simulink model "V3_sim"  (R2017a)
settings: Solver=ode45  StartTime=0.0  StopTime=Te-1  RelTol=1e-10  EnableMultiTasking=on
InitFcn:
  | clear persistent;
  | initScript;
values from neighbouring files (symbols this model uses):
  stPendel = ladePendel()    [V6_main.m]    (also in initScript.m)
  stTraj =     [Copy_of_traj.mat]    (also in traj.mat)
  T_M = .01    (= 0.01)    [initScript.m]
  x0 = [0 0 0 0]'    [RandwertproblemStates.m]    (also in initScript.m = [0 0 0 0])
settings Model: Creator=bened  LastModifiedBy=bened
settings OptimizationCC: LifeSpan=inf
settings DebuggingCC: SFUnexpectedBacktrackingDiag=warning  SFNoUnconditionalDefaultTransitionDiag=warning  SFExecutionAtInitializationDiag=none
settings GRTTargetCC: TargetLangStandard=C89/C90 (ANSI)
settings ConfigComp: CovMetricSettings=dw  CovHtmlReporting=on  CovSaveCumulativeToWorkspaceVar=on  CovSaveSingleToWorkspaceVar=on  CovExternalEMLEnable=off

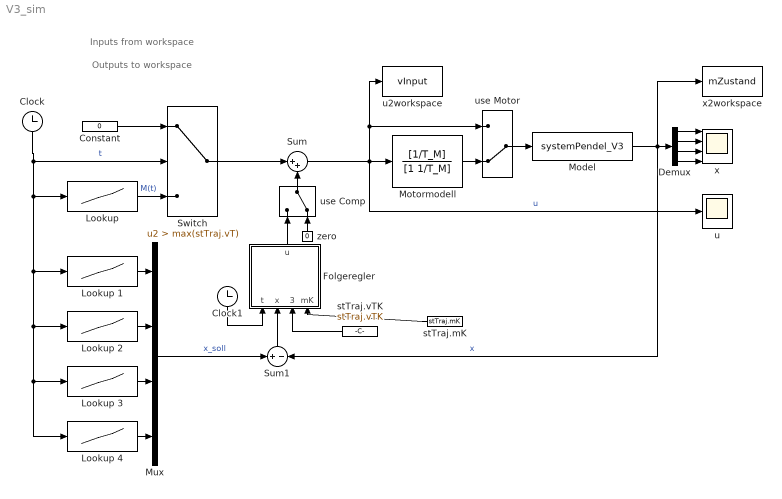
== system V3_sim ==
  note: Inputs from workspace
  note: Outputs to workspace
  Clock : Clock
  Clock1 : Clock
  Constant : Constant  Value=0
  Demux : Demux
  Folgeregler : MATLAB Function  TreatAsAtomicUnit=on
  "Lookup " : Lookup_n-D  NumberOfTableDimensions=1  LookupTableObject=lut  BreakpointsForDimension1=stTraj.vT  BreakpointsForDimension2=[1:3]  Table=stTraj.vU  InterpMethod=Cubic spline  ExtrapMethod=Clip  InternalRulePriority=Speed  RndMeth=Simplest  InputSameDT=on
  Lookup 1 : Lookup_n-D  NumberOfTableDimensions=1  LookupTableObject=lut  BreakpointsForDimension1=stTraj.vT  BreakpointsForDimension2=[1:3]  Table=stTraj.mX(1,:)  InterpMethod=Cubic spline  ExtrapMethod=Clip  InternalRulePriority=Speed  RndMeth=Simplest  InputSameDT=on
  Lookup 2 : Lookup_n-D  NumberOfTableDimensions=1  LookupTableObject=lut  BreakpointsForDimension1=stTraj.vT  BreakpointsForDimension2=[1:3]  Table=stTraj.mX(2,:)  InterpMethod=Cubic spline  ExtrapMethod=Clip  InternalRulePriority=Speed  RndMeth=Simplest  InputSameDT=on
  Lookup 3 : Lookup_n-D  NumberOfTableDimensions=1  LookupTableObject=lut  BreakpointsForDimension1=stTraj.vT  BreakpointsForDimension2=[1:3]  Table=stTraj.mX(3,:)  InterpMethod=Cubic spline  ExtrapMethod=Clip  InternalRulePriority=Speed  RndMeth=Simplest  InputSameDT=on
  Lookup 4 : Lookup_n-D  NumberOfTableDimensions=1  LookupTableObject=lut  BreakpointsForDimension1=stTraj.vT  BreakpointsForDimension2=[1:3]  Table=stTraj.mX(4,:)  InterpMethod=Cubic spline  ExtrapMethod=Clip  InternalRulePriority=Speed  RndMeth=Simplest  InputSameDT=on
  Model : M-S-Function  FunctionName=systemPendel_V3  Parameters=stPendel,x0
  Motormodell : TransferFcn  Numerator=[1/T_M]  Denominator=[1 1/T_M]
  Mux : Mux
  Sum : Sum  Inputs=|++
  Sum1 : Sum  Inputs=+|-
  Switch : Switch  Criteria=u2 > Threshold  Threshold=max(stTraj.vT)
  stTraj.mK : Constant  Value=stTraj.mK
  stTraj.vTK : Constant  Value=stTraj.vTK
  "u " : Scope
  u2workspace : ToWorkspace  VariableName=vInput  SaveFormat=Structure With Time  SampleTime=-1
  use Comp : ManualSwitch  CurrentSetting=0
  use Motor : ManualSwitch  CurrentSetting=0
  x : Scope  NumInputPorts=4
  x2workspace : ToWorkspace  VariableName=mZustand  SaveFormat=Structure With Time  SampleTime=-1
  zero : Constant  Value=0
  wires:
  Model/1 -> Sum1/2, Demux/1, x2workspace/1  "x"
  Sum/1 -> use Motor/1, u2workspace/1, Motormodell/1, "u "/1  "u"
  Demux/1 -> x/1
  Demux/2 -> x/2
  Demux/3 -> x/3
  Demux/4 -> x/4
  Clock/1 -> Lookup 4/1, Lookup 3/1, Lookup 2/1, Lookup 1/1, "Lookup "/1, Switch/2  "t"
  "Lookup "/1 -> Switch/3  "M(t)"
  Lookup 4/1 -> Mux/4
  Lookup 1/1 -> Mux/1
  Lookup 2/1 -> Mux/2
  Lookup 3/1 -> Mux/3
  Mux/1 -> Sum1/1  "x_soll"
  Sum1/1 -> Folgeregler/2(x)
  Folgeregler/1(u) -> use Comp/1
  Switch/1 -> Sum/1
  Constant/1 -> Switch/1
  Clock1/1 -> Folgeregler/1(t)
  stTraj.vTK/1 -> Folgeregler/3(vTK)
  stTraj.mK/1 -> Folgeregler/4(mK)
  Motormodell/1 -> use Motor/2
  use Comp/1 -> Sum/2
  zero/1 -> use Comp/2
  use Motor/1 -> Model/1

== matlab function V3_sim/Folgeregler ==
  data: t input; x input; u output; vTK input; mK input
function u = fcn(t,x,vTK,mK)
persistent i last;

if isempty(i)
    i = 1;
    last = length(vTK);
end

while(i<last && vTK(min([i+1, last]))<t)
    i = i+1;
end

K = mK(:,i);

u = sum(K .* x);
